simulink model "hw3_problem2"  (R2016a)
settings: Solver=VariableStepAuto  StartTime=0  StopTime=2  RelTol=1e-3
values from neighbouring files (symbols this model uses):
  bu_tot = 1    [hw3.m]
  f_d = 0    [hw3.m]
  f_sw = 10e3    (= 10000)    [hw3.m]
  kx_l = 0    [hw3.m]
  L = 1e-3    (= 0.001)    [hw3.m]
  Lambda_pm0oell = 1    [hw3.m]
  m_tot = 10e3    (= 10000)    [hw3.m]
  R = 100e-3    (= 0.1)    [hw3.m]
  V_bus = 5    [hw3.m]
libraries: dspsigops x2, cstblocks x1
settings Model: Creator=Seth Barger  LastModifiedBy=Seth Barger

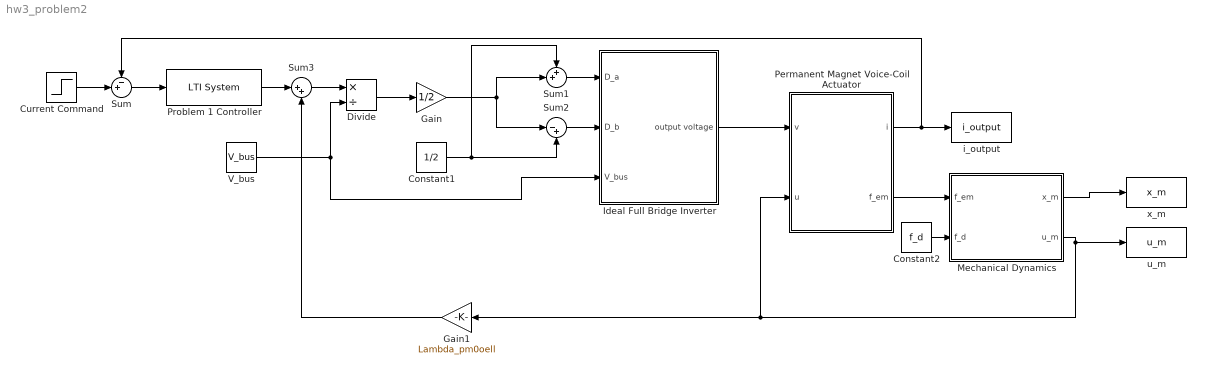
== system hw3_problem2 ==
  Constant1 : Constant  Value=1/2
  Constant2 : Constant  Value=f_d
  "Current Command " : Step  Time=0  After=5  SampleTime=0
  Divide : Product  Inputs=*/
  Gain : Gain  Gain=1/2
  Gain1 : Gain  Gain=Lambda_pm0oell
  "Ideal Full Bridge Inverter " : Subsystem
  Mechanical Dynamics : Subsystem
  Permanent Magnet Voice-Coil Actuator : Subsystem
  Problem 1 Controller : cstblocks/LTI System  sys=Gtot_elec  IC=[]
  Sum : Sum  Inputs=-+|
  Sum1 : Sum  Inputs=++|
  Sum2 : Sum  Inputs=|-+
  Sum3 : Sum  Inputs=|++
  V_bus : Constant  Value=V_bus
  i_output : ToWorkspace  VariableName=i_output  SampleTime=-1
  u_m : ToWorkspace  VariableName=u_m  SampleTime=-1
  x_m : ToWorkspace  VariableName=x_m  SampleTime=-1
  wires:
  "Ideal Full Bridge Inverter "/1(output voltage) -> Permanent Magnet Voice-Coil Actuator/1(v)
  Sum/1 -> Problem 1 Controller/1
  "Current Command "/1 -> Sum/2
  Permanent Magnet Voice-Coil Actuator/1(i) -> i_output/1, Sum/1
  Divide/1 -> Gain/1
  Gain/1 -> Sum2/1, Sum1/2
  Constant1/1 -> Sum1/1, Sum2/2
  V_bus/1 -> "Ideal Full Bridge Inverter "/3(V_bus), Divide/2
  Sum1/1 -> "Ideal Full Bridge Inverter "/1(D_a)
  Sum2/1 -> "Ideal Full Bridge Inverter "/2(D_b)
  Permanent Magnet Voice-Coil Actuator/2(f_em) -> Mechanical Dynamics/1(f_em)
  Mechanical Dynamics/2(u_m) -> u_m/1, Permanent Magnet Voice-Coil Actuator/2(u), Gain1/1
  Constant2/1 -> Mechanical Dynamics/2(f_d)
  Mechanical Dynamics/1(x_m) -> x_m/1
  Sum3/1 -> Divide/1
  Problem 1 Controller/1 -> Sum3/1
  Gain1/1 -> Sum3/2

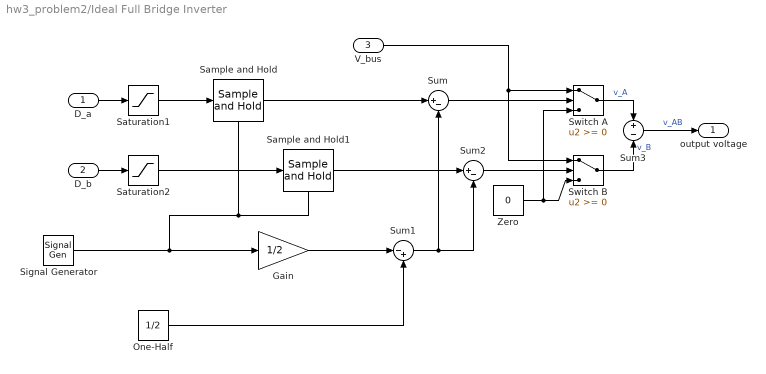
== system hw3_problem2/Ideal Full Bridge Inverter  ==
  D_a : Inport
  D_b : Inport  Port=2
  V_bus : Inport  Port=3
  Gain : Gain  Gain=1/2  SaturateOnIntegerOverflow=on  OutDataTypeStr=Inherit: Same as input  ParamDataTypeStr=Inherit: Same as input
  One-Half : Constant  Value=1/2
  Sample and Hold : dspsigops/Sample and Hold  trig=Falling edge  initCond=0  latchinput=off
  Sample and Hold1 : dspsigops/Sample and Hold  trig=Falling edge  initCond=0  latchinput=off
  Saturation1 : Saturate  UpperLimit=1  LowerLimit=0
  Saturation2 : Saturate  UpperLimit=1  LowerLimit=0
  Signal Generator : SignalGenerator  WaveForm=sawtooth  Frequency=f_sw
  Sum : Sum  Inputs=|+-  SaturateOnIntegerOverflow=on
  Sum1 : Sum  Inputs=|-+  SaturateOnIntegerOverflow=on
  Sum2 : Sum  Inputs=|+-  SaturateOnIntegerOverflow=on
  Sum3 : Sum  Inputs=+-  SaturateOnIntegerOverflow=on
  Switch A : Switch  SaturateOnIntegerOverflow=on
  Switch B : Switch  SaturateOnIntegerOverflow=on
  Zero : Constant  Value=0
  output voltage : Outport
  wires:
  Saturation2/1 -> Sample and Hold1/1
  Saturation1/1 -> Sample and Hold/1
  Sample and Hold1/1 -> Sum2/1
  D_b/1 -> Saturation2/1
  Sample and Hold/1 -> Sum/1
  D_a/1 -> Saturation1/1
  V_bus/1 -> Switch B/1, Switch A/1
  Sum1/1 -> Sum/2, Sum2/2
  Sum3/1 -> output voltage/1  "v_AB"
  Switch B/1 -> Sum3/2  "v_B"
  Switch A/1 -> Sum3/1  "v_A"
  Sum2/1 -> Switch B/2
  One-Half/1 -> Sum1/2
  Gain/1 -> Sum1/1
  Signal Generator/1 -> Gain/1, Sample and Hold1/Trigger, Sample and Hold/Trigger
  Zero/1 -> Switch B/3, Switch A/3
  Sum/1 -> Switch A/2

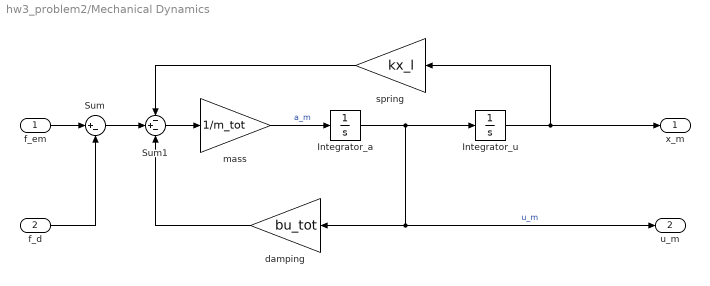
== system hw3_problem2/Mechanical Dynamics ==
  f_em : Inport
  f_d : Inport  Port=2
  Integrator_a : Integrator
  Integrator_u : Integrator
  Sum : Sum  Inputs=|+-
  Sum1 : Sum  Inputs=-+-
  damping : Gain  Gain=bu_tot
  mass : Gain  Gain=1/m_tot
  spring : Gain  Gain=kx_l
  x_m : Outport
  u_m : Outport  Port=2
  wires:
  f_em/1 -> Sum/1
  f_d/1 -> Sum/2
  mass/1 -> Integrator_a/1  "a_m"
  Integrator_a/1 -> Integrator_u/1, u_m/1, damping/1  "u_m"
  Integrator_u/1 -> x_m/1, spring/1
  Sum/1 -> Sum1/2
  Sum1/1 -> mass/1
  damping/1 -> Sum1/3
  spring/1 -> Sum1/1

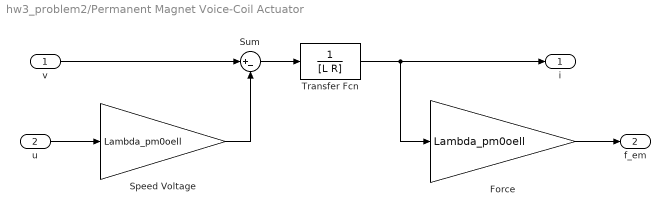
== system hw3_problem2/Permanent Magnet Voice-Coil Actuator ==
  v : Inport
  u : Inport  Port=2
  Force : Gain  Gain=Lambda_pm0oell
  Speed Voltage : Gain  Gain=Lambda_pm0oell
  Sum : Sum  Inputs=|+-
  Transfer Fcn : TransferFcn  Denominator=[L R]
  i : Outport
  f_em : Outport  Port=2
  wires:
  Transfer Fcn/1 -> i/1, Force/1
  Force/1 -> f_em/1
  v/1 -> Sum/1
  u/1 -> Speed Voltage/1
  Speed Voltage/1 -> Sum/2
  Sum/1 -> Transfer Fcn/1
